simulink model "ritminukas25str"  (R2020b)
settings: Solver=ode3  StartTime=0  StopTime=60  FixedStep=0.001  MaxStep=0.01  MinStep=0.001  RelTol=1e-3
values from neighbouring files (symbols this model uses):
  HRbasal = 118.1-0.57*amzius    [RITMINUKAS_GUI.m]    (also in ritminukas.m)
undefined symbols (not defined in the file or in its folder): Arvlm_mx, Arvlm_sp, Bmax, Dcvlm, Drsa, Kab, Kb, Kcvlm, Krsa, Ks, Peq, Pk, SIMUL, Sparas, Ssmpt, Trsa
libraries: simulink x5, simulink_extras x1
Description:
  | Heart rate (HR) regulation model encompasses three main domains: 1) heart, 2) brain – lower- and higher order neural control, and 3) vasculature.
  | The respiratory system could be interpreted as a lower-order neural control sub-domain if considered as a neural respiration center (due to link to NAmb).
  | General scheme of main HRV mechanisms – RSA (Respiration center, nucleus ambiguus (NAmb), X cranial nervus vagus, sinoatrial node (SA))
  | and baroreflexes (baroreceptors, nucleus tractus solitarius (NTS), NAmb for vagal effects; baroreceptors, NTS, rostral ventrolateral medulla (RVLM), intermediolateral column (IML) for sympathetic effects)
  | HR model itself implements the alignment of real and modeled R peaks needed for the later extraction of the residual HR variations – the displacements of the modeled R peaks relative to real R peaks – outside the model.
  | 
  | Model is intended to be managed by "Ritminukas".
  | 
  | (c) 2017-2023 Mindaugas Baranauskas
  | (c) 2020-2023 Kauno technologijos universitetas
settings Model: OrderedModelArguments=off  Creator=embar  LastModifiedBy=embar
settings SolverCC: AlgebraicLoopSolver=LineSearch  AutoInsertRateTranBlk=on
settings DebuggingCC: ReadBeforeWriteMsg=DisableAll  WriteAfterWriteMsg=DisableAll  WriteAfterReadMsg=DisableAll  InheritedTsInSrcMsg=none  MultiTaskDSMMsg=none  ArithmeticOperatorsInVariantConditions=warning
settings HardwareCC: ProdBitPerLong=64  ProdHWDeviceType=Intel->x86-64 (Linux 64)
settings ModelReferenceCC: UpdateModelReferenceTargets=IfOutOfDate
settings SFSimCC: SFSimEcho=off  SimUseLocalCustomCode=off  CustomCodeUndefinedFunction=UseInterfaceOnly
settings RTWCC: RTWUseLocalCustomCode=off

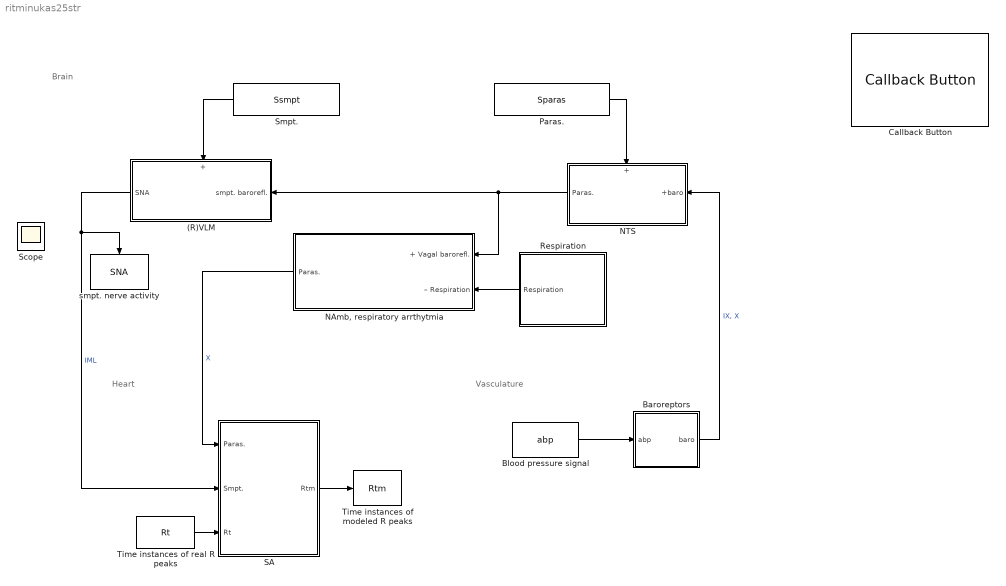
== system ritminukas25str ==
  note: Vasculature
  note: Brain
  note: Heart
  (R)VLM : Subsystem
      settings: PortSchema="{\"entries\":[{\"content\":{\"sides\":[{\"content\":{\"connectorIds\":[\"In1\"]},\"type\":\"ConnectorPlacement.EquallySpacedRectSide\",\"uuid\":\"2587094f-5909-4e4d-adae-6e37e468e632\"},{\"content\":{\"connectorIds\":[],\"side\":\"RIGHT\"},\"type\":\"ConnectorPlacement.EquallySpacedRectSide\",\"uuid\":\"5adc800e-be50-4960-b6ce-292c95efe34b\"},{\"content\":{\"connectorIds\":[\"Out1\"],\"side\":\"TOP\"},\"type\":\"ConnectorPlacement.EquallySpacedRectSide\",\"uuid\":\"1273915d-836a-40db-a65c-184b4676baca\"},{\"content\":{\"connectorIds\":[\"In2\"],\"side\":\"BOTTOM\"},\"type\":\"ConnectorPlacement.EquallySpacedRectSide\",\"uuid\":\"fee847fd-6d03-4e6a-997d-0ae8ebef8894\"},{\"content\":{\"connectorIds\":[],\"side\":\"HIDDEN\"},\"type\":\"ConnectorPlacement.EquallySpacedRectSide\",\"uuid\":\"96feea81-bcd9-434e-ba31-ce0f8d5ce338\"}]},\"type\":\"ConnectorPlacement.EquallySpacedConnector\",\"uuid\":\"71bc25ff-42d1-4af8-bd56-0239d3b58f9c\"}],\"packageUris\":[\"http://schema.mathworks.com/mf0/Connector/R2020b\"],\"version\":\"1.0\"}"
  Baroreptors : Subsystem
  Blood pressure signal : FromWorkspace  VariableName=abp  OutDataTypeStr=double  SampleTime=-1  Interpolate=off  ZeroCross=off  OutputAfterFinalValue=Holding final value
  Callback Button : CallbackButton  ButtonText=Atverti Ritminuką
      settings: ClickFcn=RITMINUKAS_GUI
  "NAmb, respiratory arrthytmia" : Subsystem
  NTS : Subsystem
      settings: PortSchema="{\"entries\":[{\"content\":{\"sides\":[{\"content\":{\"connectorIds\":[\"In1\"]},\"type\":\"ConnectorPlacement.EquallySpacedRectSide\",\"uuid\":\"56d02fb8-b640-4ea2-971f-8a590660cfa9\"},{\"content\":{\"connectorIds\":[\"Out1\"],\"side\":\"RIGHT\"},\"type\":\"ConnectorPlacement.EquallySpacedRectSide\",\"uuid\":\"2953568c-9b61-4620-8ffa-2ce1f3e0db66\"},{\"content\":{\"connectorIds\":[\"In2\"],\"side\":\"TOP\"},\"type\":\"ConnectorPlacement.EquallySpacedRectSide\",\"uuid\":\"0760ba7c-0f98-4f7d-9569-d549d317009c\"},{\"content\":{\"connectorIds\":[],\"side\":\"HIDDEN\"},\"type\":\"ConnectorPlacement.EquallySpacedRectSide\",\"uuid\":\"a596e4f4-b606-4dbe-87d3-cc75ce852313\"}]},\"type\":\"ConnectorPlacement.EquallySpacedConnector\",\"uuid\":\"474f6ead-aa07-4e28-bb2e-f9df4ff82bcb\"}],\"packageUris\":[\"http://schema.mathworks.com/mf0/Connector/R2020b\"],\"version\":\"1.0\"}"
  Paras. : Constant  Value=Sparas
  Respiration : Subsystem
  SA : Subsystem
  Smpt. : Constant  Value=Ssmpt
  Time instances of modeled R peaks : ToWorkspace  VariableName=Rtm  SaveFormat=Timeseries  SampleTime=-1
  Time instances of real R peaks : FromWorkspace  VariableName=Rt  OutDataTypeStr=double  SampleTime=-1  Interpolate=off  ZeroCross=off  OutputAfterFinalValue=Holding final value
  smpt. nerve activity : ToWorkspace  VariableName=SNA  SaveFormat=Timeseries  SampleTime=-1
  Scope : Scope
  wires:
  Paras./1 -> NTS/2(+)
  Respiration/1(Respiration) -> "NAmb, respiratory arrthytmia"/2(– Respiration)
  Blood pressure signal/1 -> Baroreptors/1(abp)
  Baroreptors/1(baro) -> NTS/1(+baro)  "IX, X"
  "NAmb, respiratory arrthytmia"/1(Paras.) -> SA/1(Paras.)  "X"
  (R)VLM/1(SNA) -> SA/2(Smpt.), smpt. nerve activity/1  "IML"
  Smpt./1 -> (R)VLM/1(+)
  Time instances of real R peaks/1 -> SA/3(Rt)
  SA/1(Rtm) -> Time instances of modeled R peaks/1
  NTS/1(Paras.) -> (R)VLM/2(smpt. barorefl.), "NAmb, respiratory arrthytmia"/1(+ Vagal barorefl.)

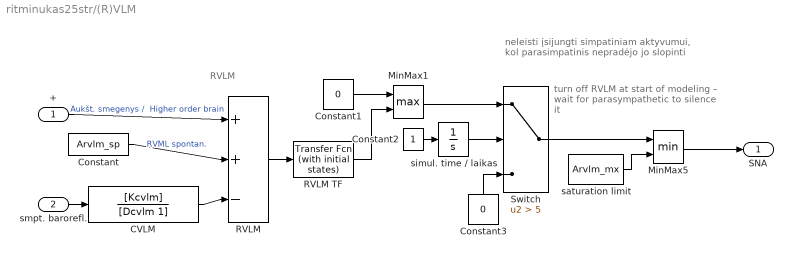
== system ritminukas25str/(R)VLM ==
  note: RVLM
  note: turn off RVLM at start of modeling –
      | wait for parasympathetic to silence it
  note: neleisti įsijungti simpatiniam aktyvumui,
      |  kol parasimpatinis nepradėjo jo slopinti
  + : Inport
  smpt. barorefl. : Inport  Port=2
  CVLM : TransferFcn  Numerator=[Kcvlm]  Denominator=[Dcvlm 1]
  Constant : Constant  Value=Arvlm_sp
  Constant1 : Constant  Value=0
  Constant2 : Constant
  Constant3 : Constant  Value=0
  MinMax1 : MinMax  Function=max  Inputs=2
  MinMax5 : MinMax  Inputs=2
  RVLM : Sum  Inputs=++|-  OutMin=0  OutDataTypeStr=double
  RVLM TF : simulink_extras/Additional Linear/Transfer Fcn (with initial states)  N=1  D=[0.1 1]  X0=0
  Switch : Switch  Criteria=u2 > Threshold  Threshold=5
  saturation limit : Constant  Value=Arvlm_mx
  simul. time / laikas : Integrator
  SNA : Outport
  wires:
  Constant1/1 -> MinMax1/1
  RVLM TF/1 -> MinMax1/2
  RVLM/1 -> RVLM TF/1
  +/1 -> RVLM/1  "Aukšt. smegenys /  Higher order brain"
  MinMax1/1 -> Switch/1
  Constant2/1 -> simul. time / laikas/1
  simul. time / laikas/1 -> Switch/2
  Constant3/1 -> Switch/3
  saturation limit/1 -> MinMax5/2
  Switch/1 -> MinMax5/1
  MinMax5/1 -> SNA/1
  smpt. barorefl./1 -> CVLM/1
  CVLM/1 -> RVLM/3
  Constant/1 -> RVLM/2  "RVML spontan."

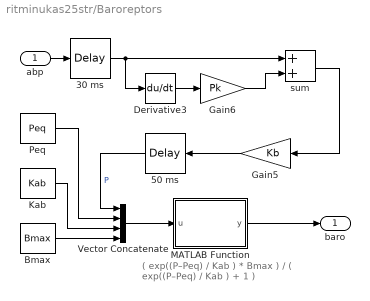
== system ritminukas25str/Baroreptors ==
  note: ( exp((P–Peq) /  Kab ) * Bmax ) /
      | ( exp((P–Peq) /  Kab ) + 1 )
  abp : Inport
  30 ms : TransportDelay  DelayTime=0.03  InitialOutput=Peq
  50 ms : TransportDelay  DelayTime=0.05  InitialOutput=Peq
  Bmax : Constant  Value=Bmax
  Derivative3 : Derivative
  Gain5 : Gain  Gain=Kb
  Gain6 : Gain  Gain=Pk
  Kab : Constant  Value=Kab
  MATLAB Function : MATLAB Function  TreatAsAtomicUnit=on
  Peq : Constant  Value=Peq
  Vector Concatenate : Concatenate  NumInputs=4
  sum : Sum
  baro : Outport  VectorParamsAs1DForOutWhenUnconnected=off
  wires:
  Gain5/1 -> 50 ms/1
  Vector Concatenate/1 -> MATLAB Function/1(u)
  MATLAB Function/1(y) -> baro/1
  50 ms/1 -> Vector Concatenate/1  "P"
  Derivative3/1 -> Gain6/1
  Kab/1 -> Vector Concatenate/3
  Gain6/1 -> sum/2
  Bmax/1 -> Vector Concatenate/4
  sum/1 -> Gain5/1
  Peq/1 -> Vector Concatenate/2
  abp/1 -> 30 ms/1
  30 ms/1 -> sum/1, Derivative3/1

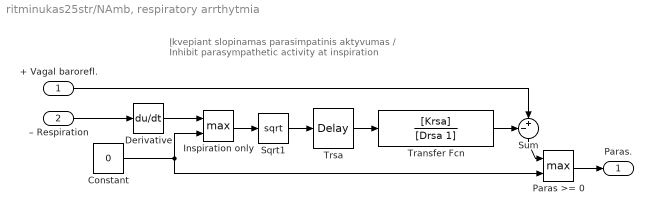
== system ritminukas25str/NAmb, respiratory arrthytmia ==
  note: Įkvepiant slopinamas parasimpatinis aktyvumas /
      | Inhibit parasympathetic activity at inspiration
  + Vagal barorefl. : Inport
  – Respiration : Inport  Port=2
  Constant : Constant  Value=0
  Derivative : Derivative
  Inspiration only : MinMax  Function=max  Inputs=2
  Paras >= 0 : MinMax  Function=max  Inputs=2
  Sqrt1 : Sqrt  SaturateOnIntegerOverflow=on
  Sum : Sum  Inputs=-+|  OutMin=0
  Transfer Fcn : TransferFcn  Numerator=[Krsa]  Denominator=[Drsa 1]
  Trsa : TransportDelay  DelayTime=Trsa  BufferSize=8192
  Paras. : Outport  VectorParamsAs1DForOutWhenUnconnected=off
  wires:
  + Vagal barorefl./1 -> Sum/2
  Sum/1 -> Paras >= 0/1
  Transfer Fcn/1 -> Sum/1
  Derivative/1 -> Inspiration only/1
  – Respiration/1 -> Derivative/1
  Sqrt1/1 -> Trsa/1
  Constant/1 -> Inspiration only/2, Paras >= 0/2
  Inspiration only/1 -> Sqrt1/1
  Paras >= 0/1 -> Paras./1
  Trsa/1 -> Transfer Fcn/1

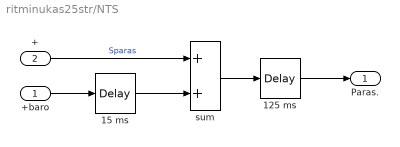
== system ritminukas25str/NTS ==
  +baro : Inport
  + : Inport  Port=2
  125 ms : TransportDelay  DelayTime=0.125  InitialOutput=Sparas
  15 ms : TransportDelay  DelayTime=0.015
  sum : Sum
  Paras. : Outport
  wires:
  15 ms/1 -> sum/2
  +/1 -> sum/1  "Sparas"
  sum/1 -> 125 ms/1
  +baro/1 -> 15 ms/1
  125 ms/1 -> Paras./1

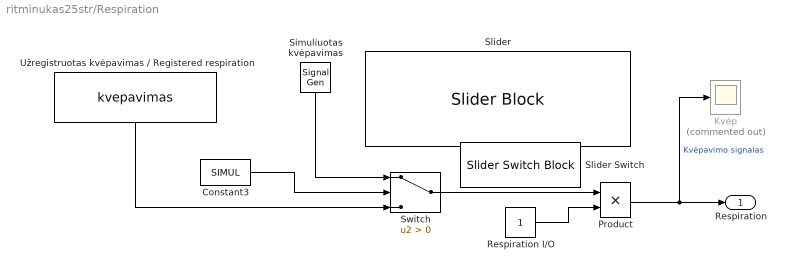
== system ritminukas25str/Respiration ==
  Constant3 : Constant  Value=SIMUL
  Kvėp : Scope  Commented=on
  Product : Product
  Respiration I/O : Constant
  Simuliuotas kvėpavimas : SignalGenerator  Amplitude=0.5  Frequency=0.1  VectorParams1D=off
  Slider : SliderBlock  ScaleMax=0.4  TickInterval=0.1
  Slider Switch : SliderSwitchBlock  LabelPosition=Hide
      settings: Values={{'O', 'I'}, [0 1]}
  Switch : Switch  Criteria=u2 > Threshold
  Užregistruotas kvėpavimas / Registered respiration : FromWorkspace  VariableName=kvepavimas  OutDataTypeStr=double  SampleTime=-1  ZeroCross=off  OutputAfterFinalValue=Holding final value
  Respiration : Outport  VectorParamsAs1DForOutWhenUnconnected=off
  wires:
  Užregistruotas kvėpavimas / Registered respiration/1 -> Switch/3
  Simuliuotas kvėpavimas/1 -> Switch/1
  Respiration I/O/1 -> Product/2
  Product/1 -> Kvėp/1, Respiration/1  "Kvėpavimo signalas"
  Constant3/1 -> Switch/2
  Switch/1 -> Product/1

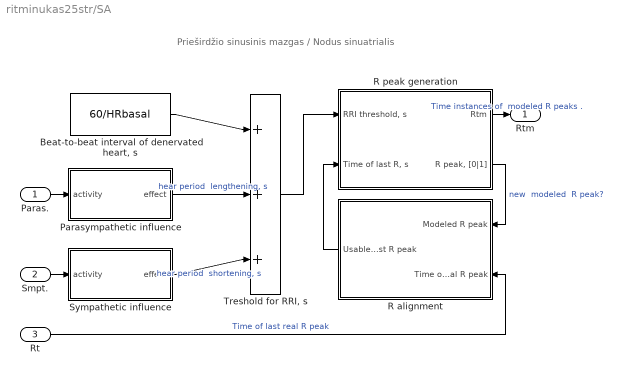
== system ritminukas25str/SA ==
  note: Prieširdžio sinusinis mazgas / Nodus sinuatrialis
  Paras. : Inport
  Smpt. : Inport  Port=2
  Rt : Inport  Port=3
  "Beat-to-beat interval of denervated heart, s " : Constant  Value=60/HRbasal
  Parasympathetic influence : Subsystem
  R alignment : Subsystem
  R peak generation : Subsystem
  Sympathetic influence : Subsystem
  "Treshold for RRI, s" : Sum  Inputs=+|+|+
  Rtm : Outport
  wires:
  Paras./1 -> Parasympathetic influence/1(activity)
  Parasympathetic influence/1(effect) -> "Treshold for RRI, s"/2  "hear period  lengthening, s"
  Sympathetic influence/1(effect) -> "Treshold for RRI, s"/3  "hear period  shortening, s"
  "Beat-to-beat interval of denervated heart, s "/1 -> "Treshold for RRI, s"/1
  "Treshold for RRI, s"/1 -> R peak generation/1("RRI threshold, s")
  Smpt./1 -> Sympathetic influence/1(activity)
  Rt/1 -> R alignment/2(Time of last real R peak)  "Time of last real R peak"
  R alignment/1(Usable time of last R peak) -> R peak generation/2("Time of last R, s")
  R peak generation/2("R peak, [0|1]") -> R alignment/1(Modeled R peak)  "new  modeled  R peak?"
  R peak generation/1(Rtm) -> Rtm/1  "Time instances of  modeled R peaks ."

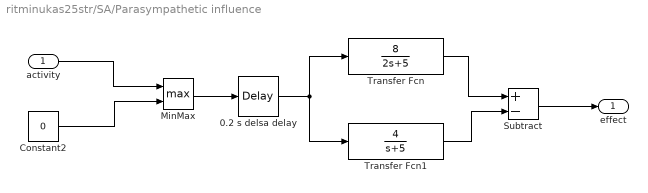
== system ritminukas25str/SA/Parasympathetic influence ==
  activity : Inport
  0.2 s delsa delay : TransportDelay  DelayTime=0.2
  Constant2 : Constant  Value=0
  MinMax : MinMax  Function=max  Inputs=2  RndMeth=Zero
  Subtract : Sum  Inputs=+-
  Transfer Fcn : TransferFcn  Numerator=8  Denominator=[2 5]
  Transfer Fcn1 : TransferFcn  Numerator=4  Denominator=[1 5]
  effect : Outport  VectorParamsAs1DForOutWhenUnconnected=off
  wires:
  activity/1 -> MinMax/1
  Transfer Fcn/1 -> Subtract/1
  Subtract/1 -> effect/1
  Transfer Fcn1/1 -> Subtract/2
  0.2 s delsa delay/1 -> Transfer Fcn/1, Transfer Fcn1/1
  Constant2/1 -> MinMax/2
  MinMax/1 -> 0.2 s delsa delay/1

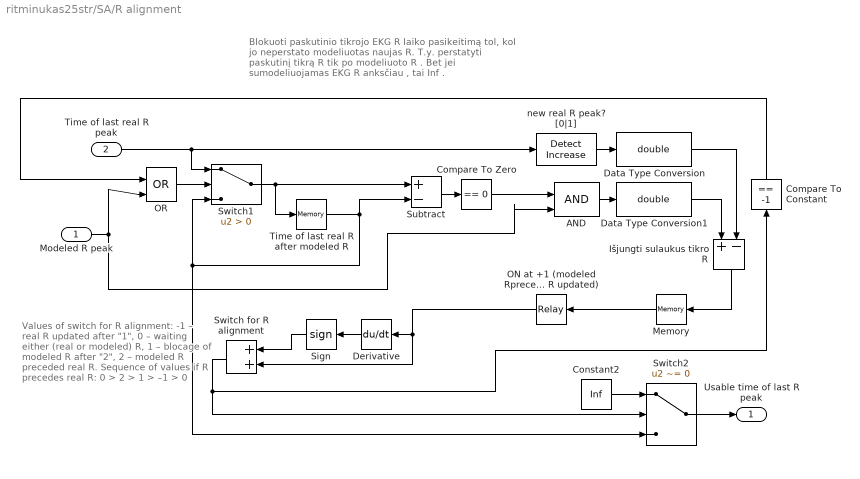
== system ritminukas25str/SA/R alignment ==
  note: Values of switch for R alignment:
      | -1 – real R updated after "1",
      | 0 – waiting either (real or modeled) R,
      | 1 – blocage of modeled R after "2",
      | 2 – modeled R preceded real R.
      | Sequence of values
      | if R precedes real R:
      | 0 > 2 > 1 > –1 > 0
  note: Blokuoti paskutinio tikrojo EKG R laiko pasikeitimą tol,
      | kol jo neperstato modeliuotas naujas R. T.y.
      | perstatyti paskutinį tikrą R tik po modeliuoto R .
      | Bet jei sumodeliuojamas EKG R anksčiau , tai Inf .
  Modeled R peak : Inport
  Time of last real R peak : Inport  Port=2
  AND : Logic  IconShape=distinctive  AllPortsSameDT=off  OutDataTypeStr=boolean
  Compare To Constant : simulink/Logic and Bit Operations/Compare To Constant  relop===  const=-1  OutDataTypeStr=boolean
  Compare To Zero : simulink/Logic and Bit Operations/Compare To Zero  relop===  OutDataTypeStr=boolean
  Constant2 : Constant  Value=Inf
  Data Type Conversion : DataTypeConversion  OutDataTypeStr=double
  Data Type Conversion1 : DataTypeConversion  OutDataTypeStr=double
  Derivative : Derivative
  Išjungti sulaukus tikro R : Sum  Inputs=+-  InputSameDT=on
  Memory : Memory
  "ON at +1 (modeled Rpreceded real R), OFF at –1 (real R updated)" : Relay  OnSwitchValue=1  OffSwitchValue=-1
  OR : Logic  Operator=OR  IconShape=distinctive  AllPortsSameDT=off  OutDataTypeStr=boolean
  Sign : Signum
  Subtract : Sum  Inputs=+-
  Switch for R alignment : Sum  InputSameDT=on
  Switch1 : Switch  Criteria=u2 > Threshold
  Switch2 : Switch  Criteria=u2 ~= 0
  Time of last real R after modeled R : Memory  InitialCondition=NaN
  new real R peak? [0|1] : simulink/Logic and Bit Operations/Detect Increase  vinit=0  OutDataTypeStr=boolean
  Usable time of last R peak : Outport
  wires:
  Switch1/1 -> Subtract/1, Time of last real R after modeled R/1
  Modeled R peak/1 -> OR/2, AND/2
  Time of last real R peak/1 -> new real R peak? [0|1]/1, Switch1/1
  Time of last real R after modeled R/1 -> Switch1/3, Switch2/3, Subtract/2
  "ON at +1 (modeled Rpreceded real R), OFF at –1 (real R updated)"/1 -> Switch for R alignment/2, Derivative/1
  Compare To Constant/1 -> OR/1
  Sign/1 -> Switch for R alignment/1
  Data Type Conversion/1 -> Išjungti sulaukus tikro R/2
  Subtract/1 -> Compare To Zero/1
  AND/1 -> Data Type Conversion1/1
  Compare To Zero/1 -> AND/1
  Data Type Conversion1/1 -> Išjungti sulaukus tikro R/1
  OR/1 -> Switch1/2
  Memory/1 -> "ON at +1 (modeled Rpreceded real R), OFF at –1 (real R updated)"/1
  Išjungti sulaukus tikro R/1 -> Memory/1
  Derivative/1 -> Sign/1
  new real R peak? [0|1]/1 -> Data Type Conversion/1
  Switch for R alignment/1 -> Switch2/2, Compare To Constant/1
  Switch2/1 -> Usable time of last R peak/1
  Constant2/1 -> Switch2/1

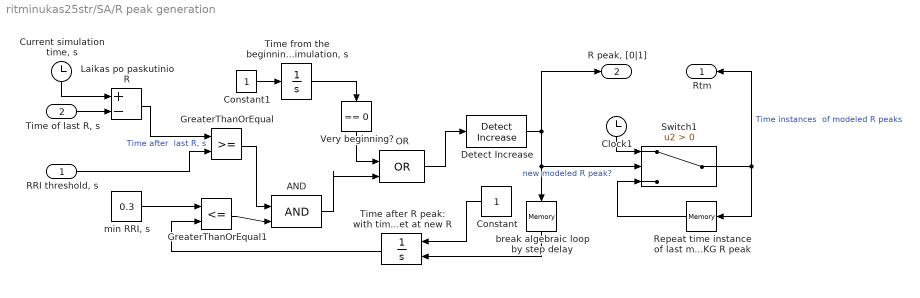
== system ritminukas25str/SA/R peak generation ==
  "RRI threshold, s" : Inport
  "Time of last R, s" : Inport  Port=2
  AND : Logic  IconShape=distinctive  AllPortsSameDT=off  OutDataTypeStr=boolean
  Clock1 : Clock
  Constant : Constant
  Constant1 : Constant
  "Current simulation time, s" : Clock
  Detect Increase : simulink/Logic and Bit Operations/Detect Increase  vinit=0  OutDataTypeStr=boolean
  GreaterThanOrEqual : RelationalOperator  OutDataTypeStr=boolean  RndMeth=Simplest
  GreaterThanOrEqual1 : RelationalOperator  Operator=<=  OutDataTypeStr=boolean  RndMeth=Simplest
  Laikas po paskutinio R : Sum  Inputs=+-
  OR : Logic  Operator=OR  IconShape=distinctive  AllPortsSameDT=off  OutDataTypeStr=boolean
  Repeat time instance of last modeled EKG R peak : Memory  InitialCondition=NaN
  Switch1 : Switch  Criteria=u2 > Threshold
  Time after R peak: with timer reset at new R : Integrator  ExternalReset=either  UpperSaturationLimit=1  LowerSaturationLimit=0
  "Time from the beginning of simulation, s" : Integrator
  Very beginning? : simulink/Logic and Bit Operations/Compare To Zero  relop===  OutDataTypeStr=boolean
  break algebraic loop by step delay : Memory
  "min RRI, s" : Constant  Value=0.3  OutDataTypeStr=Inherit: Inherit via back propagation
  Rtm : Outport
  "R peak, [0|1]" : Outport  Port=2
  wires:
  Constant1/1 -> "Time from the beginning of simulation, s"/1
  "Time from the beginning of simulation, s"/1 -> Very beginning?/1
  GreaterThanOrEqual/1 -> AND/1
  GreaterThanOrEqual1/1 -> AND/2
  Very beginning?/1 -> OR/1
  Clock1/1 -> Switch1/1
  "Current simulation time, s"/1 -> Laikas po paskutinio R/1
  Laikas po paskutinio R/1 -> GreaterThanOrEqual/1  "Time after  last R, s"
  OR/1 -> Detect Increase/1
  AND/1 -> OR/2
  Constant/1 -> Time after R peak: with timer reset at new R/1
  Time after R peak: with timer reset at new R/1 -> GreaterThanOrEqual1/2
  Switch1/1 -> Rtm/1, Repeat time instance of last modeled EKG R peak/1  "Time instances  of modeled R peaks"
  break algebraic loop by step delay/1 -> Time after R peak: with timer reset at new R/2
  Repeat time instance of last modeled EKG R peak/1 -> Switch1/3
  "min RRI, s"/1 -> GreaterThanOrEqual1/1
  "RRI threshold, s"/1 -> GreaterThanOrEqual/2
  "Time of last R, s"/1 -> Laikas po paskutinio R/2
  Detect Increase/1 -> "R peak, [0|1]"/1, Switch1/2, break algebraic loop by step delay/1  "new modeled R peak?"

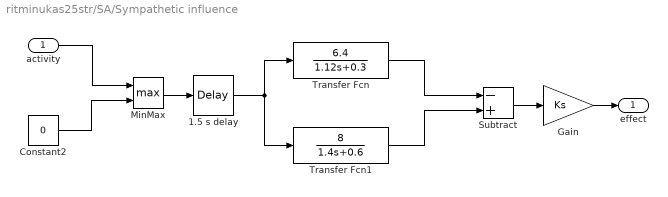
== system ritminukas25str/SA/Sympathetic influence ==
  activity : Inport
  1.5 s delay : TransportDelay  DelayTime=1.5  BufferSize=2048
  Constant2 : Constant  Value=0
  Gain : Gain  Gain=Ks
  MinMax : MinMax  Function=max  Inputs=2  RndMeth=Zero
  Subtract : Sum  Inputs=-+
  Transfer Fcn : TransferFcn  Numerator=6.4  Denominator=[1.12 0.3]
  Transfer Fcn1 : TransferFcn  Numerator=8  Denominator=[1.4 0.6]
  effect : Outport  VectorParamsAs1DForOutWhenUnconnected=off
  wires:
  Transfer Fcn/1 -> Subtract/1
  activity/1 -> MinMax/1
  1.5 s delay/1 -> Transfer Fcn1/1, Transfer Fcn/1
  Transfer Fcn1/1 -> Subtract/2
  Constant2/1 -> MinMax/2
  MinMax/1 -> 1.5 s delay/1
  Subtract/1 -> Gain/1
  Gain/1 -> effect/1

== matlab function ritminukas25str/Baroreptors/MATLAB Function ==
  data: u input; y output
function y = fcn(u)
% ( exp((P–Peq) /  Kab ) * Bmax ) / ( exp((P–Peq) /  Kab ) + 1 ) 

y = (exp((u(1) - u(2)  ) /  u(3) ) * u(4) + 0)  /  (exp((u(1) - u(2)  ) /   u(3)) +1 ) ;
